simulink model "ece456hw82b"  (R2017b)
settings: Solver=VariableStepAuto  StartTime=0.0  StopTime=10.0  RelTol=1e-3
values from neighbouring files (symbols this model uses):
  Ki = .1    (= 0.1)    [ece456hw7.m]    (also in ece456hw8.m = 3)
  Kp = 1.65    [ece456hw7.m]    (also in ece456hw8.m = 14.8603130573)
settings Model: Creator=b  LastModifiedBy=b

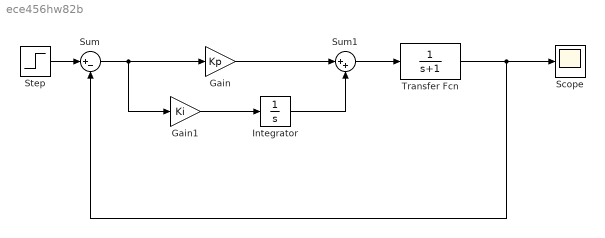
== system ece456hw82b ==
  Gain : Gain  Gain=Kp
  Gain1 : Gain  Gain=Ki
  Integrator : Integrator
  Scope : Scope
  Step : Step  SampleTime=0
  Sum : Sum  Inputs=|+-
  Sum1 : Sum  Inputs=|++
  Transfer Fcn : TransferFcn  Denominator=[1 1]
  wires:
  Step/1 -> Sum/1
  Transfer Fcn/1 -> Sum/2, Scope/1
  Sum1/1 -> Transfer Fcn/1
  Sum/1 -> Gain1/1, Gain/1
  Gain/1 -> Sum1/1
  Gain1/1 -> Integrator/1
  Integrator/1 -> Sum1/2
